simulink model "controlModel"  (R2015a)
settings: Solver=ode45  StartTime=0.0  StopTime=50  RelTol=1e-3
undefined symbols (not defined in the file): i
settings Model: Creator=jinkale  LastModifiedBy=jinkale

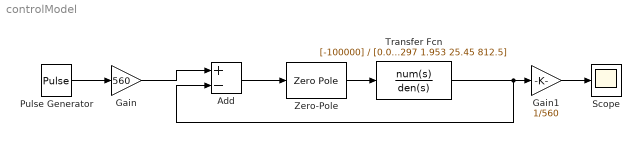
== system controlModel ==
  Add : Sum  Inputs=+-
  Gain : Gain  Gain=560
  Gain1 : Gain  Gain=1/560
  Pulse Generator : DiscretePulseGenerator  PulseType=Time based  Amplitude=3  Period=10  PulseWidth=50
  Scope : Scope
      settings: TimeRange=50  YMin=0.02  YMax=0.034  MaxDataPoints=500000
  Transfer Fcn : TransferFcn  Numerator=[-100000]  Denominator=[0.0297 1.953 25.45 812.5]
  Zero-Pole : ZeroPole  Zeros=[3.0405+i*12.6,3.0405-i*12.6]  Poles=[0 -200]  Gain=[-0.038702]
  wires:
  Pulse Generator/1 -> Gain/1
  Gain/1 -> Add/1
  Add/1 -> Zero-Pole/1
  Zero-Pole/1 -> Transfer Fcn/1
  Transfer Fcn/1 -> Gain1/1, Add/2
  Gain1/1 -> Scope/1
